simulink model "wabs_perceptionmodel_VPT_Limbic_v3_adj"  (R2014b)
settings: Solver=ode3  StartTime=0.0  StopTime=r.t(end)  FixedStep=z.dt  MaxStep=0.01  RelTol=1e-3
undefined symbols (not defined in the file or in its folder): G0, G0_hat, r, z
libraries: vrlib x3, dspinverses x1
settings Model: Creator=dpool  LastModifiedBy=fdrop
settings DataIOCC: SignalLoggingSaveFormat=ModelDataLogs
settings OptimizationCC: ExpressionDepthLimit=2147483647
settings DebuggingCC: AlgebraicLoopMsg=none  UnderspecifiedInitializationDetection=Classic  MergeDetectMultiDrivingBlocksExec=none  FcnCallInpInsideContextMsg=EnableAllAsWarning  StateNameClashWarn=warning  InitInArrayFormatMsg=none
settings SFSimCC: SimParseCustomCode=off
settings GRTTargetCC: CombineOutputUpdateFcns=off  GRTInterface=on

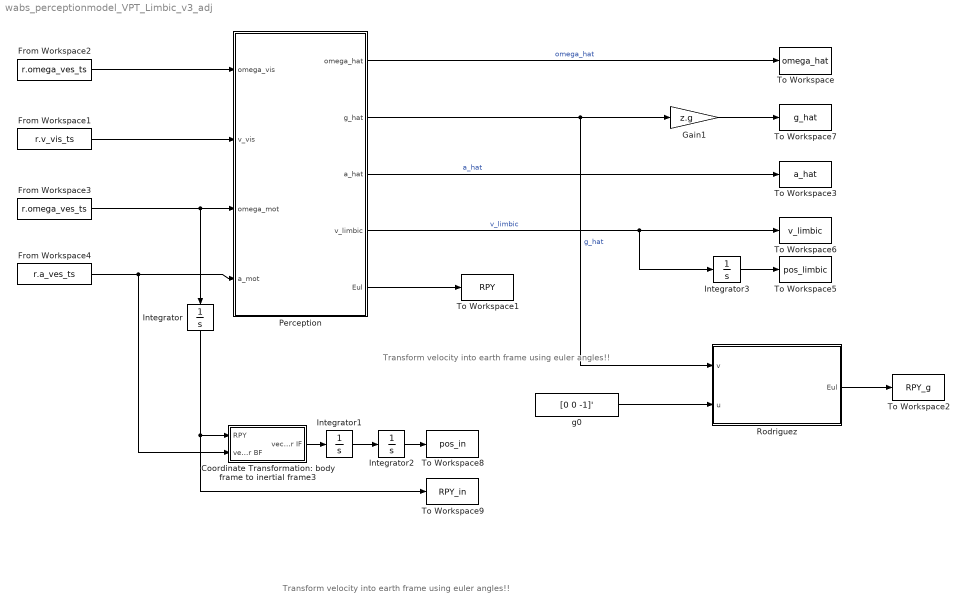
== system wabs_perceptionmodel_VPT_Limbic_v3_adj ==
  note: Transform velocity into earth frame using euler angles!!
  note: Transform velocity into earth frame using euler angles!!
  Coordinate Transformation: body frame to inertial frame3 : Subsystem
  From Workspace1 : FromWorkspace  VariableName=r.v_vis_ts  SampleTime=0
  From Workspace2 : FromWorkspace  VariableName=r.omega_ves_ts  SampleTime=0
  From Workspace3 : FromWorkspace  VariableName=r.omega_ves_ts  SampleTime=0
  From Workspace4 : FromWorkspace  VariableName=r.a_ves_ts  SampleTime=0
  Gain1 : Gain  Gain=z.g
  Integrator{,1..3} (4 alike) : Integrator
  Perception : Subsystem  mask{G0_mot=[0; 0; -1]}
      mask TypeOptions G0_mot:
      | Input Selection & Kinematics/Initial orientation,
      | motion/Value
  Rodriguez : MATLAB Function  TreatAsAtomicUnit=on
  To Workspace : ToWorkspace  VariableName=omega_hat  SampleTime=-1
  To Workspace1 : ToWorkspace  VariableName=RPY  SampleTime=-1
  To Workspace2 : ToWorkspace  VariableName=RPY_g  SampleTime=-1
  To Workspace3 : ToWorkspace  VariableName=a_hat  SampleTime=-1
  To Workspace5 : ToWorkspace  VariableName=pos_limbic  SampleTime=-1
  To Workspace6 : ToWorkspace  VariableName=v_limbic  SampleTime=-1
  To Workspace7 : ToWorkspace  VariableName=g_hat  SampleTime=-1
  To Workspace8 : ToWorkspace  VariableName=pos_in  SampleTime=-1
  To Workspace9 : ToWorkspace  VariableName=RPY_in  SampleTime=-1
  g0 : Constant  Value=[0 0 -1]'
  wires:
  Perception/1(omega_hat) -> To Workspace/1  "omega_hat"
  Perception/2(g_hat) -> Rodriguez/1(v), Gain1/1  "g_hat"
  Perception/3(a_hat) -> To Workspace3/1  "a_hat"
  Perception/4(v_limbic) -> Integrator3/1, To Workspace6/1  "v_limbic"
  Gain1/1 -> To Workspace7/1
  From Workspace4/1 -> Coordinate Transformation: body frame to inertial frame3/2(vector BF), Perception/4(a_mot)
  From Workspace3/1 -> Integrator/1, Perception/3(omega_mot)
  Perception/5(Eul) -> To Workspace1/1
  From Workspace1/1 -> Perception/2(v_vis)
  From Workspace2/1 -> Perception/1(omega_vis)
  Integrator3/1 -> To Workspace5/1
  Integrator/1 -> To Workspace9/1, Coordinate Transformation: body frame to inertial frame3/1(RPY)
  Coordinate Transformation: body frame to inertial frame3/1(vector IF) -> Integrator1/1
  Integrator1/1 -> Integrator2/1
  Integrator2/1 -> To Workspace8/1
  g0/1 -> Rodriguez/2(u)
  Rodriguez/1(Eul) -> To Workspace2/1

== system wabs_perceptionmodel_VPT_Limbic_v3_adj/Coordinate Transformation: body frame to inertial frame3 ==
  RPY : Inport
  vector BF : Inport  Port=2
  Body2Inertial : MATLAB Function  TreatAsAtomicUnit=on
  Product : Product  Multiplication=Matrix(*)  RndMeth=Zero
  vector IF : Outport
  wires:
  Body2Inertial/1(DCM) -> Product/1
  RPY/1 -> Body2Inertial/1(RPY)
  Product/1 -> vector IF/1
  vector BF/1 -> Product/2

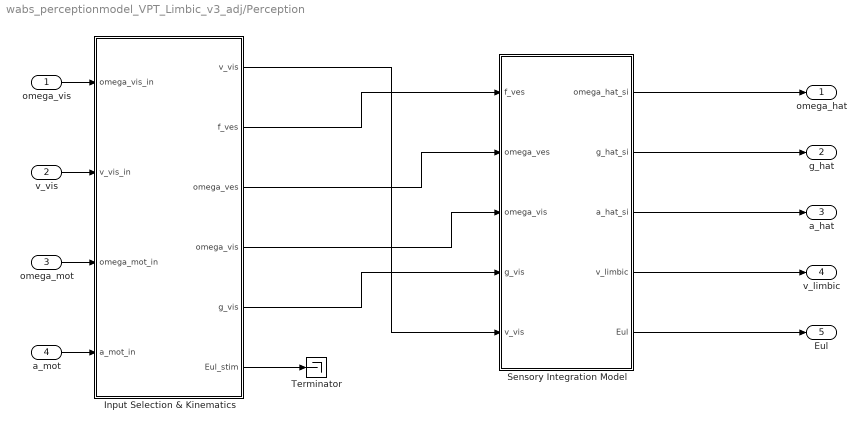
== system wabs_perceptionmodel_VPT_Limbic_v3_adj/Perception ==
  omega_vis : Inport
  v_vis : Inport  Port=2
  omega_mot : Inport  Port=3
  a_mot : Inport  Port=4
  Input Selection & Kinematics : Subsystem
  Sensory Integration Model : Subsystem
  Terminator : Terminator
  omega_hat : Outport
  g_hat : Outport  Port=2
  a_hat : Outport  Port=3
  v_limbic : Outport  Port=4
  Eul : Outport  Port=5
  wires:
  Input Selection & Kinematics/5(g_vis) -> Sensory Integration Model/4(g_vis)
  Input Selection & Kinematics/4(omega_vis) -> Sensory Integration Model/3(omega_vis)
  Input Selection & Kinematics/3(omega_ves) -> Sensory Integration Model/2(omega_ves)
  Input Selection & Kinematics/2(f_ves) -> Sensory Integration Model/1(f_ves)
  Input Selection & Kinematics/1(v_vis) -> Sensory Integration Model/5(v_vis)
  Sensory Integration Model/1(omega_hat_si) -> omega_hat/1
  omega_vis/1 -> Input Selection & Kinematics/1(omega_vis_in)
  Sensory Integration Model/2(g_hat_si) -> g_hat/1
  v_vis/1 -> Input Selection & Kinematics/2(v_vis_in)
  omega_mot/1 -> Input Selection & Kinematics/3(omega_mot_in)
  Sensory Integration Model/3(a_hat_si) -> a_hat/1
  a_mot/1 -> Input Selection & Kinematics/4(a_mot_in)
  Sensory Integration Model/4(v_limbic) -> v_limbic/1
  Sensory Integration Model/5(Eul) -> Eul/1
  Input Selection & Kinematics/6(Eul_stim) -> Terminator/1

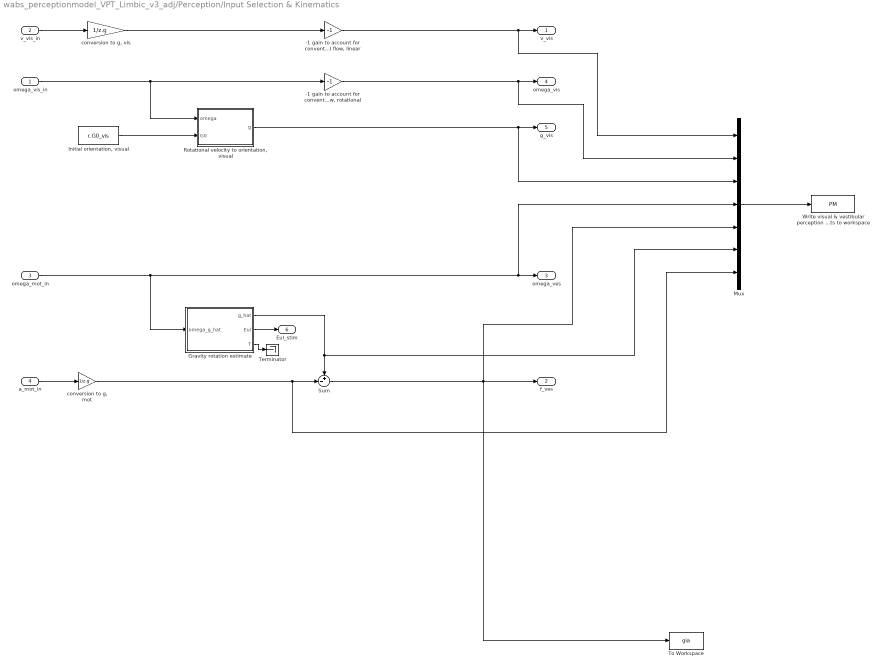
== system wabs_perceptionmodel_VPT_Limbic_v3_adj/Perception/Input Selection & Kinematics ==
  omega_vis_in : Inport
  v_vis_in : Inport  Port=2
  omega_mot_in : Inport  Port=3
  a_mot_in : Inport  Port=4
  "-1 gain to account for convention in visual flow, linear" : Gain  Gain=-1
  "-1 gain to account for convention in visual flow, rotational" : Gain  Gain=-1
  Gravity rotation estimate : Subsystem
  "Initial orientation, visual" : Constant  Value=r.G0_vis
  Mux : Mux  Inputs=7
  "Rotational velocity to orientation, visual" : Subsystem
  Sum : Sum  Inputs=+-|
  Terminator : Terminator
  To Workspace : ToWorkspace  VariableName=gia  SampleTime=-1
  Write visual & vestibular perception model inputs to workspace : ToWorkspace  VariableName=PM  SampleTime=-1
  "conversion to g, mot" : Gain  Gain=1/z.g
  "conversion to g, vis" : Gain  Gain=1/z.g
  v_vis : Outport
  f_ves : Outport  Port=2
  omega_ves : Outport  Port=3
  omega_vis : Outport  Port=4
  g_vis : Outport  Port=5
  Eul_stim : Outport  Port=6
  wires:
  a_mot_in/1 -> "conversion to g, mot"/1
  "-1 gain to account for convention in visual flow, linear"/1 -> v_vis/1, Mux/1
  v_vis_in/1 -> "conversion to g, vis"/1
  omega_vis_in/1 -> "-1 gain to account for convention in visual flow, rotational"/1, "Rotational velocity to orientation, visual"/1(omega)
  "Rotational velocity to orientation, visual"/1(g) -> g_vis/1, Mux/3
  "Initial orientation, visual"/1 -> "Rotational velocity to orientation, visual"/2(G0)
  "-1 gain to account for convention in visual flow, rotational"/1 -> omega_vis/1, Mux/2
  omega_mot_in/1 -> Gravity rotation estimate/1(omega_g_hat), omega_ves/1, Mux/4
  Gravity rotation estimate/1(g_hat) -> Sum/1, Mux/6
  Mux/1 -> Write visual & vestibular perception model inputs to workspace/1
  "conversion to g, vis"/1 -> "-1 gain to account for convention in visual flow, linear"/1
  "conversion to g, mot"/1 -> Sum/2, Mux/7
  Sum/1 -> To Workspace/1, f_ves/1, Mux/5
  Gravity rotation estimate/2(Eul) -> Eul_stim/1
  Gravity rotation estimate/3(T) -> Terminator/1

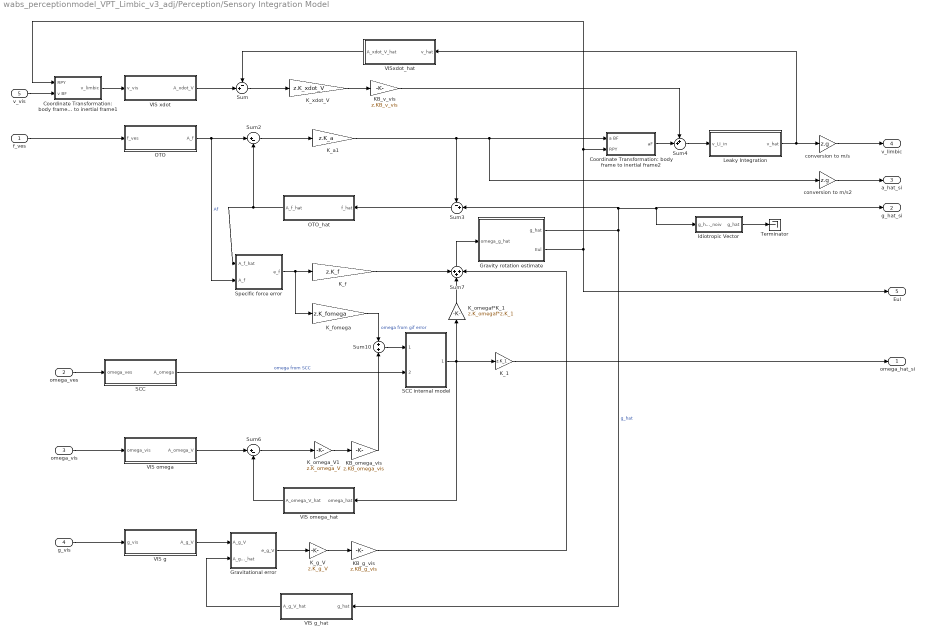
== system wabs_perceptionmodel_VPT_Limbic_v3_adj/Perception/Sensory Integration Model ==
  f_ves : Inport
  omega_ves : Inport  Port=2
  omega_vis : Inport  Port=3
  g_vis : Inport  Port=4
  v_vis : Inport  Port=5
  Coordinate Transformation: body frame to inertial frame1 : Subsystem
  Coordinate Transformation: body frame to inertial frame2 : Subsystem
  Gravitational error : Subsystem
  Gravity rotation estimate : Subsystem
  Idiotropic Vector : Subsystem
  KB_g_vis : Gain  Gain=z.KB_g_vis
  KB_omega_vis : Gain  Gain=z.KB_omega_vis
  KB_v_vis : Gain  Gain=z.KB_v_vis
  K_1 : Gain  Gain=z.K_1
  K_a1 : Gain  Gain=z.K_a
  K_f : Gain  Gain=z.K_f
  K_fomega : Gain  Gain=z.K_fomega
  K_g_V : Gain  Gain=z.K_g_V
  K_omega_V1 : Gain  Gain=z.K_omega_V
  K_omegaf*K_1 : Gain  Gain=z.K_omegaf*z.K_1
  K_xdot_V : Gain  Gain=z.K_xdot_V
  Leaky Integration : Subsystem
  OTO : Subsystem
  OTO_hat : Subsystem
  SCC : Subsystem
  SCC internal model : Subsystem
  Specific force error : Subsystem
  Sum : Sum  Inputs=-+|
  Sum10 : Sum
  Sum2 : Sum  Inputs=|+-
  Sum3 : Sum  Inputs=-+|
  Sum4 : Sum  Inputs=++|
  Sum6 : Sum  Inputs=|+-
  Sum7 : Sum  Inputs=+++
  Terminator : Terminator
  VIS g : Subsystem
  VIS g_hat : Subsystem
  VIS omega : Subsystem
  VIS omega_hat : Subsystem
  VIS xdot : Subsystem
  VISxdot_hat : Subsystem
  conversion to m/s : Gain  Gain=z.g
  conversion to m/s2 : Gain  Gain=z.g
  omega_hat_si : Outport
  g_hat_si : Outport  Port=2
  a_hat_si : Outport  Port=3
  v_limbic : Outport  Port=4
  Eul : Outport  Port=5
  wires:
  Sum2/1 -> K_a1/1
  OTO/1(A_f) -> Sum2/1, Specific force error/2(A_f)  "Af"
  Sum3/1 -> OTO_hat/1(f_hat)
  SCC/1(A_omega) -> SCC internal model/2(omega_SCC)  "omega from SCC"
  OTO_hat/1(A_f_hat) -> Sum2/2, Specific force error/1(A_f_hat)
  Gravity rotation estimate/1(g_hat) -> Idiotropic Vector/1(g_hat_noiv), g_hat_si/1, Sum3/2, VIS g_hat/1(g_hat)  "g_hat"
  Specific force error/1(e_f) -> K_f/1, K_fomega/1
  K_fomega/1 -> Sum10/1  "omega from gif error"
  VIS xdot/1(A_xdot_V) -> Sum/2
  VISxdot_hat/1(A_xdot_V_hat) -> Sum/1
  Sum/1 -> K_xdot_V/1
  K_xdot_V/1 -> KB_v_vis/1
  VIS omega/1(A_omega_V) -> Sum6/1
  Sum6/1 -> K_omega_V1/1
  VIS omega_hat/1(A_omega_V_hat) -> Sum6/2
  VIS g/1(A_g_V) -> Gravitational error/1(A_g_V)
  Gravitational error/1(e_g_V) -> K_g_V/1
  VIS g_hat/1(A_g_V_hat) -> Gravitational error/2(A_g_V_hat)
  K_1/1 -> omega_hat_si/1
  K_g_V/1 -> KB_g_vis/1
  K_omega_V1/1 -> KB_omega_vis/1
  Leaky Integration/1(v_hat) -> VISxdot_hat/1(v_hat), conversion to m/s/1
  Sum7/1 -> Gravity rotation estimate/1(omega_g_hat)
  f_ves/1 -> OTO/1(f_ves)
  omega_ves/1 -> SCC/1(omega_ves)
  omega_vis/1 -> VIS omega/1(omega_vis)
  g_vis/1 -> VIS g/1(g_vis)
  KB_g_vis/1 -> Sum7/3
  conversion to m/s/1 -> v_limbic/1
  conversion to m/s2/1 -> a_hat_si/1
  K_f/1 -> Sum7/1
  K_omegaf*K_1/1 -> Sum7/2
  K_a1/1 -> Sum3/1, Coordinate Transformation: body frame to inertial frame2/1(a BF), conversion to m/s2/1
  Idiotropic Vector/1(g_hat) -> Terminator/1
  v_vis/1 -> Coordinate Transformation: body frame to inertial frame1/2(v BF)
  Coordinate Transformation: body frame to inertial frame1/1(v_limbic) -> VIS xdot/1(v_vis)
  Gravity rotation estimate/2(Eul) -> Coordinate Transformation: body frame to inertial frame2/2(RPY), Coordinate Transformation: body frame to inertial frame1/1(RPY), Eul/1
  Coordinate Transformation: body frame to inertial frame2/1(aF) -> Sum4/2
  Sum4/1 -> Leaky Integration/1(v_LI_in)
  KB_v_vis/1 -> Sum4/1
  KB_omega_vis/1 -> Sum10/2
  Sum10/1 -> SCC internal model/1(omega_vis+GIF)
  SCC internal model/1(omega_hat) -> K_1/1, VIS omega_hat/1(omega_hat), K_omegaf*K_1/1

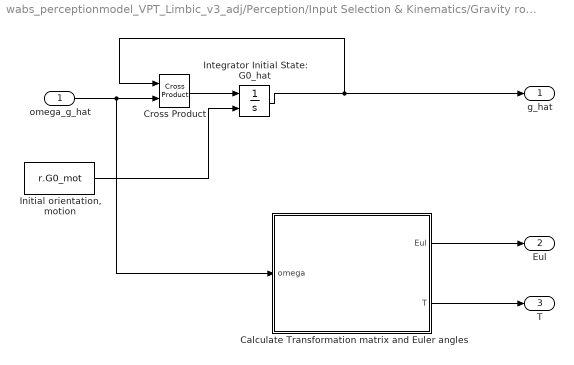
== system wabs_perceptionmodel_VPT_Limbic_v3_adj/Perception/Input Selection & Kinematics/Gravity rotation estimate ==
  omega_g_hat : Inport
  Calculate Transformation matrix and Euler angles : Subsystem
  Cross Product : vrlib/Utilities/Cross Product
  "Initial orientation, motion" : Constant  Value=r.G0_mot
  Integrator Initial State: G0_hat : Integrator  InitialConditionSource=external  InitialCondition=G0_hat
  g_hat : Outport
  Eul : Outport  Port=2
  T : Outport  Port=3
  wires:
  Integrator Initial State: G0_hat/1 -> Cross Product/1, g_hat/1
  Cross Product/1 -> Integrator Initial State: G0_hat/1
  omega_g_hat/1 -> Calculate Transformation matrix and Euler angles/1(omega), Cross Product/2
  Calculate Transformation matrix and Euler angles/1(Eul) -> Eul/1
  Calculate Transformation matrix and Euler angles/2(T) -> T/1
  "Initial orientation, motion"/1 -> Integrator Initial State: G0_hat/2

== system wabs_perceptionmodel_VPT_Limbic_v3_adj/Perception/Input Selection & Kinematics/Rotational velocity to orientation, visual ==
  omega : Inport
  G0 : Inport  Port=2
  Cross Product : vrlib/Utilities/Cross Product
  Integrator : Integrator  InitialConditionSource=external  InitialCondition=G0
  Normalize vector1 : Subsystem
  g : Outport
  wires:
  Integrator/1 -> Normalize vector1/1(G), Cross Product/1
  Cross Product/1 -> Integrator/1
  Normalize vector1/1(g) -> g/1
  omega/1 -> Cross Product/2
  G0/1 -> Integrator/2

== system wabs_perceptionmodel_VPT_Limbic_v3_adj/Perception/Sensory Integration Model/Coordinate Transformation: body frame to inertial frame1 ==
  RPY : Inport
  v BF : Inport  Port=2
  Body2Inertial : MATLAB Function  TreatAsAtomicUnit=on
  Product : Product  Multiplication=Matrix(*)  RndMeth=Zero
  v_limbic : Outport
  wires:
  Body2Inertial/1(DCM) -> Product/1
  RPY/1 -> Body2Inertial/1(RPY)
  Product/1 -> v_limbic/1
  v BF/1 -> Product/2

== system wabs_perceptionmodel_VPT_Limbic_v3_adj/Perception/Sensory Integration Model/Coordinate Transformation: body frame to inertial frame2 ==
  a BF : Inport
  RPY : Inport  Port=2
  Body2Inertial : MATLAB Function  TreatAsAtomicUnit=on
  Product : Product  Multiplication=Matrix(*)  RndMeth=Zero
  aF : Outport
  wires:
  a BF/1 -> Product/2
  Product/1 -> aF/1
  RPY/1 -> Body2Inertial/1(RPY)
  Body2Inertial/1(DCM) -> Product/1

== system wabs_perceptionmodel_VPT_Limbic_v3_adj/Perception/Sensory Integration Model/Gravitational error ==
  A_g_V : Inport
  A_g_V_hat : Inport  Port=2
  MATLAB Function : MATLAB Function  TreatAsAtomicUnit=on
  e_g_V : Outport
  wires:
  A_g_V/1 -> MATLAB Function/1(g)
  A_g_V_hat/1 -> MATLAB Function/2(g_hat)
  MATLAB Function/1(e_g) -> e_g_V/1

== system wabs_perceptionmodel_VPT_Limbic_v3_adj/Perception/Sensory Integration Model/Gravity rotation estimate ==
  omega_g_hat : Inport
  Calculate Euler angles from omega CLEANER : Subsystem
  Cross Product : vrlib/Utilities/Cross Product
  Integrator Initial State: G0_hat : Integrator  InitialCondition=r.G0_hat
  g_hat : Outport
  Eul : Outport  Port=2
  wires:
  Integrator Initial State: G0_hat/1 -> Cross Product/1, g_hat/1
  Cross Product/1 -> Integrator Initial State: G0_hat/1
  omega_g_hat/1 -> Calculate Euler angles from omega CLEANER/1(omega), Cross Product/2
  Calculate Euler angles from omega CLEANER/1(Eul) -> Eul/1

== system wabs_perceptionmodel_VPT_Limbic_v3_adj/Perception/Sensory Integration Model/Idiotropic Vector ==
  g_hat_noiv : Inport
  Idiotropic vector: constant unity vector aligned with vertical body axis : Constant  Value=r.G_iv
  K_iv : Gain  Gain=z.K_iv
  Normalize vector : Subsystem
  Sum : Sum  Inputs=++|
  g_hat : Outport
  wires:
  Normalize vector/1(g) -> g_hat/1
  Idiotropic vector: constant unity vector aligned with vertical body axis/1 -> K_iv/1
  K_iv/1 -> Sum/1
  g_hat_noiv/1 -> Sum/2
  Sum/1 -> Normalize vector/1(G)

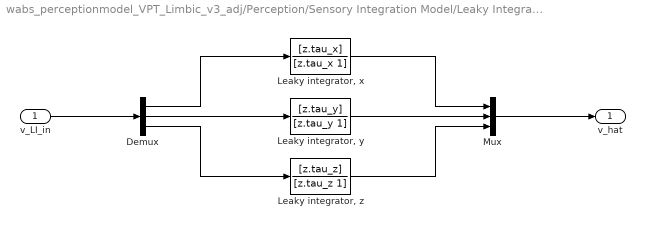
== system wabs_perceptionmodel_VPT_Limbic_v3_adj/Perception/Sensory Integration Model/Leaky Integration ==
  v_LI_in : Inport
  Demux : Demux  Outputs=3
  "Leaky integrator, x" : TransferFcn  Numerator=[z.tau_x]  Denominator=[z.tau_x 1]
  "Leaky integrator, y" : TransferFcn  Numerator=[z.tau_y]  Denominator=[z.tau_y 1]
  "Leaky integrator, z" : TransferFcn  Numerator=[z.tau_z]  Denominator=[z.tau_z 1]
  Mux : Mux  Inputs=3
  v_hat : Outport
  wires:
  v_LI_in/1 -> Demux/1
  Mux/1 -> v_hat/1
  "Leaky integrator, y"/1 -> Mux/2
  Demux/2 -> "Leaky integrator, y"/1
  Demux/1 -> "Leaky integrator, x"/1
  "Leaky integrator, x"/1 -> Mux/1
  Demux/3 -> "Leaky integrator, z"/1
  "Leaky integrator, z"/1 -> Mux/3

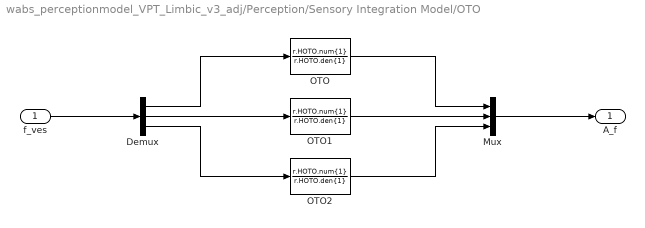
== system wabs_perceptionmodel_VPT_Limbic_v3_adj/Perception/Sensory Integration Model/OTO ==
  f_ves : Inport
  Demux : Demux  Outputs=3
  Mux : Mux  Inputs=3
  OTO : TransferFcn  Numerator=r.HOTO.num{1}  Denominator=r.HOTO.den{1}
  OTO1 : TransferFcn  Numerator=r.HOTO.num{1}  Denominator=r.HOTO.den{1}
  OTO2 : TransferFcn  Numerator=r.HOTO.num{1}  Denominator=r.HOTO.den{1}
  A_f : Outport
  wires:
  f_ves/1 -> Demux/1
  Mux/1 -> A_f/1
  OTO1/1 -> Mux/2
  Demux/2 -> OTO1/1
  Demux/1 -> OTO/1
  OTO/1 -> Mux/1
  Demux/3 -> OTO2/1
  OTO2/1 -> Mux/3

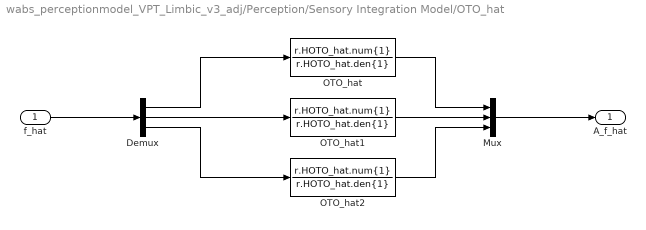
== system wabs_perceptionmodel_VPT_Limbic_v3_adj/Perception/Sensory Integration Model/OTO_hat ==
  f_hat : Inport
  Demux : Demux  Outputs=3
  Mux : Mux  Inputs=3
  OTO_hat : TransferFcn  Numerator=r.HOTO_hat.num{1}  Denominator=r.HOTO_hat.den{1}
  OTO_hat1 : TransferFcn  Numerator=r.HOTO_hat.num{1}  Denominator=r.HOTO_hat.den{1}
  OTO_hat2 : TransferFcn  Numerator=r.HOTO_hat.num{1}  Denominator=r.HOTO_hat.den{1}
  A_f_hat : Outport
  wires:
  f_hat/1 -> Demux/1
  Mux/1 -> A_f_hat/1
  OTO_hat1/1 -> Mux/2
  Demux/2 -> OTO_hat1/1
  Demux/1 -> OTO_hat/1
  OTO_hat/1 -> Mux/1
  Demux/3 -> OTO_hat2/1
  OTO_hat2/1 -> Mux/3

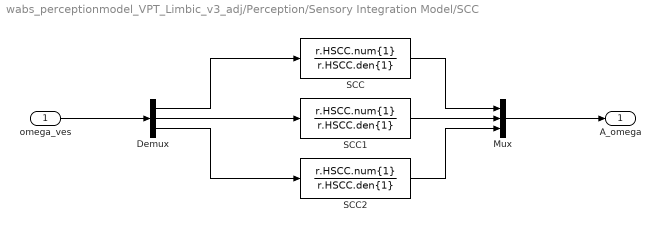
== system wabs_perceptionmodel_VPT_Limbic_v3_adj/Perception/Sensory Integration Model/SCC ==
  omega_ves : Inport
  Demux : Demux  Outputs=3
  Mux : Mux  Inputs=3
  SCC : TransferFcn  Numerator=r.HSCC.num{1}  Denominator=r.HSCC.den{1}
  SCC1 : TransferFcn  Numerator=r.HSCC.num{1}  Denominator=r.HSCC.den{1}
  SCC2 : TransferFcn  Numerator=r.HSCC.num{1}  Denominator=r.HSCC.den{1}
  A_omega : Outport
  wires:
  omega_ves/1 -> Demux/1
  Mux/1 -> A_omega/1
  SCC1/1 -> Mux/2
  Demux/2 -> SCC1/1
  Demux/1 -> SCC/1
  SCC/1 -> Mux/1
  Demux/3 -> SCC2/1
  SCC2/1 -> Mux/3

== system wabs_perceptionmodel_VPT_Limbic_v3_adj/Perception/Sensory Integration Model/SCC internal model ==
  omega_vis+GIF : Inport
  omega_SCC : Inport  Port=2
  K_omega : Gain  Gain=z.K_omega
  SCC_hat : Subsystem
  Sum5 : Sum
  omega_hat : Outport
  wires:
  omega_SCC/1 -> K_omega/1
  SCC_hat/1(A_omega_hat) -> omega_hat/1
  omega_vis+GIF/1 -> Sum5/1
  K_omega/1 -> Sum5/2
  Sum5/1 -> SCC_hat/1(omega_hat)

== system wabs_perceptionmodel_VPT_Limbic_v3_adj/Perception/Sensory Integration Model/Specific force error ==
  A_f_hat : Inport
  A_f : Inport  Port=2
  Specific force rotation error : MATLAB Function  TreatAsAtomicUnit=on
  e_f : Outport
  wires:
  Specific force rotation error/1(ef) -> e_f/1
  A_f/1 -> Specific force rotation error/1(af)
  A_f_hat/1 -> Specific force rotation error/2(af_hat)

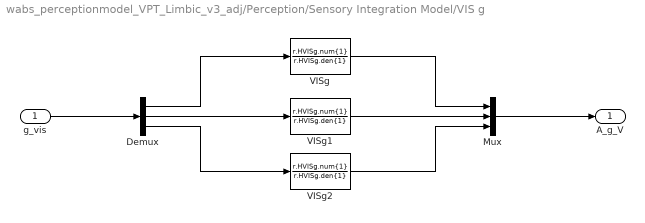
== system wabs_perceptionmodel_VPT_Limbic_v3_adj/Perception/Sensory Integration Model/VIS g ==
  g_vis : Inport
  Demux : Demux  Outputs=3
  Mux : Mux  Inputs=3
  VISg : TransferFcn  Numerator=r.HVISg.num{1}  Denominator=r.HVISg.den{1}
  VISg1 : TransferFcn  Numerator=r.HVISg.num{1}  Denominator=r.HVISg.den{1}
  VISg2 : TransferFcn  Numerator=r.HVISg.num{1}  Denominator=r.HVISg.den{1}
  A_g_V : Outport
  wires:
  g_vis/1 -> Demux/1
  Mux/1 -> A_g_V/1
  VISg1/1 -> Mux/2
  Demux/2 -> VISg1/1
  Demux/1 -> VISg/1
  VISg/1 -> Mux/1
  Demux/3 -> VISg2/1
  VISg2/1 -> Mux/3

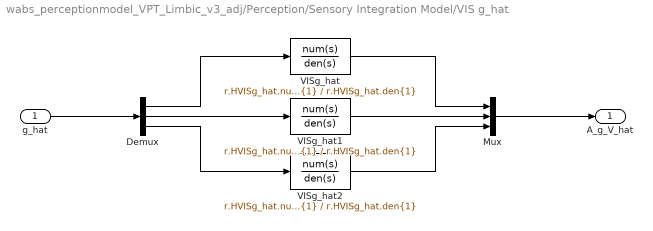
== system wabs_perceptionmodel_VPT_Limbic_v3_adj/Perception/Sensory Integration Model/VIS g_hat ==
  g_hat : Inport
  Demux : Demux  Outputs=3
  Mux : Mux  Inputs=3
  VISg_hat : TransferFcn  Numerator=r.HVISg_hat.num{1}  Denominator=r.HVISg_hat.den{1}
  VISg_hat1 : TransferFcn  Numerator=r.HVISg_hat.num{1}  Denominator=r.HVISg_hat.den{1}
  VISg_hat2 : TransferFcn  Numerator=r.HVISg_hat.num{1}  Denominator=r.HVISg_hat.den{1}
  A_g_V_hat : Outport
  wires:
  g_hat/1 -> Demux/1
  Mux/1 -> A_g_V_hat/1
  VISg_hat1/1 -> Mux/2
  Demux/2 -> VISg_hat1/1
  Demux/1 -> VISg_hat/1
  VISg_hat/1 -> Mux/1
  Demux/3 -> VISg_hat2/1
  VISg_hat2/1 -> Mux/3

== system wabs_perceptionmodel_VPT_Limbic_v3_adj/Perception/Sensory Integration Model/VIS omega ==
  omega_vis : Inport
  Demux : Demux  Outputs=3
  Mux : Mux  Inputs=3
  VISomega : TransferFcn  Numerator=r.HVISomega.num{1}  Denominator=r.HVISomega.den{1}
  VISomega1 : TransferFcn  Numerator=r.HVISomega.num{1}  Denominator=r.HVISomega.den{1}
  VISomega2 : TransferFcn  Numerator=r.HVISomega.num{1}  Denominator=r.HVISomega.den{1}
  A_omega_V : Outport
  wires:
  omega_vis/1 -> Demux/1
  Mux/1 -> A_omega_V/1
  VISomega1/1 -> Mux/2
  Demux/2 -> VISomega1/1
  Demux/1 -> VISomega/1
  VISomega/1 -> Mux/1
  Demux/3 -> VISomega2/1
  VISomega2/1 -> Mux/3

== system wabs_perceptionmodel_VPT_Limbic_v3_adj/Perception/Sensory Integration Model/VIS omega_hat ==
  omega_hat : Inport
  Demux : Demux  Outputs=3
  Mux : Mux  Inputs=3
  VISomega_hat : TransferFcn  Numerator=r.HVISomega_hat.num{1}  Denominator=r.HVISomega_hat.den{1}
  VISomega_hat1 : TransferFcn  Numerator=r.HVISomega_hat.num{1}  Denominator=r.HVISomega_hat.den{1}
  VISomega_hat2 : TransferFcn  Numerator=r.HVISomega_hat.num{1}  Denominator=r.HVISomega_hat.den{1}
  A_omega_V_hat : Outport
  wires:
  omega_hat/1 -> Demux/1
  Mux/1 -> A_omega_V_hat/1
  VISomega_hat1/1 -> Mux/2
  Demux/2 -> VISomega_hat1/1
  Demux/1 -> VISomega_hat/1
  VISomega_hat/1 -> Mux/1
  Demux/3 -> VISomega_hat2/1
  VISomega_hat2/1 -> Mux/3

== system wabs_perceptionmodel_VPT_Limbic_v3_adj/Perception/Sensory Integration Model/VIS xdot ==
  v_vis : Inport
  Demux : Demux  Outputs=3
  Mux : Mux  Inputs=3
  VISxdot : TransferFcn  Numerator=r.HVISxdot.num{1}  Denominator=r.HVISxdot.den{1}
  VISxdot1 : TransferFcn  Numerator=r.HVISxdot.num{1}  Denominator=r.HVISxdot.den{1}
  VISxdot2 : TransferFcn  Numerator=r.HVISxdot.num{1}  Denominator=r.HVISxdot.den{1}
  A_xdot_V : Outport
  wires:
  v_vis/1 -> Demux/1
  Mux/1 -> A_xdot_V/1
  VISxdot1/1 -> Mux/2
  Demux/2 -> VISxdot1/1
  Demux/1 -> VISxdot/1
  VISxdot/1 -> Mux/1
  Demux/3 -> VISxdot2/1
  VISxdot2/1 -> Mux/3

== system wabs_perceptionmodel_VPT_Limbic_v3_adj/Perception/Sensory Integration Model/VISxdot_hat ==
  v_hat : Inport
  Demux : Demux  Outputs=3
  Mux : Mux  Inputs=3
  VISxdot_hat : TransferFcn  Numerator=r.HVISxdot_hat.num{1}  Denominator=r.HVISxdot_hat.den{1}
  VISxdot_hat1 : TransferFcn  Numerator=r.HVISxdot_hat.num{1}  Denominator=r.HVISxdot_hat.den{1}
  VISxdot_hat2 : TransferFcn  Numerator=r.HVISxdot_hat.num{1}  Denominator=r.HVISxdot_hat.den{1}
  A_xdot_V_hat : Outport
  wires:
  v_hat/1 -> Demux/1
  Mux/1 -> A_xdot_V_hat/1
  VISxdot_hat1/1 -> Mux/2
  Demux/2 -> VISxdot_hat1/1
  Demux/1 -> VISxdot_hat/1
  VISxdot_hat/1 -> Mux/1
  Demux/3 -> VISxdot_hat2/1
  VISxdot_hat2/1 -> Mux/3

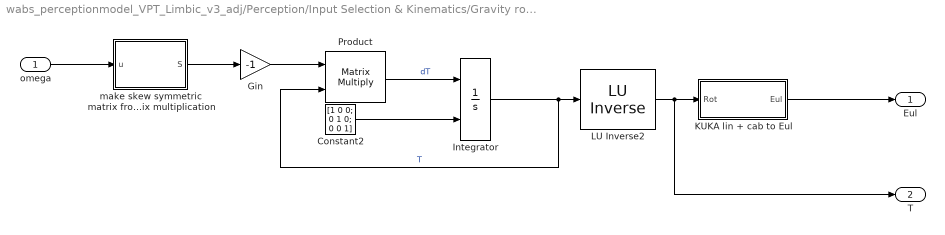
== system wabs_perceptionmodel_VPT_Limbic_v3_adj/Perception/Input Selection & Kinematics/Gravity rotation estimate/Calculate Transformation matrix and Euler angles ==
  omega : Inport
  " LU Inverse2" : dspinverses/ LU Inverse
  Constant2 : Constant  Value=[1 0 0; 0 1 0; 0 0 1]
  Gin : Gain  Gain=-1
  Integrator : Integrator  InitialConditionSource=external  InitialCondition=[1 0 0; 0 1 0; 0 0 1]
  KUKA lin + cab to Eul : Subsystem  AncestorBlock=KUKA_Control_libs/KUKA lin + cab to Eul
  Product : Product  Multiplication=Matrix(*)
  make skew symmetric matrix from omega for matrix multiplication : MATLAB Function  TreatAsAtomicUnit=on
  Eul : Outport
  T : Outport  Port=2
  wires:
  Integrator/1 -> " LU Inverse2"/1, Product/2  "T"
  KUKA lin + cab to Eul/1(Eul) -> Eul/1
  make skew symmetric matrix from omega for matrix multiplication/1(S) -> Gin/1
  Product/1 -> Integrator/1  "dT"
  omega/1 -> make skew symmetric matrix from omega for matrix multiplication/1(u)
  Constant2/1 -> Integrator/2
  Gin/1 -> Product/1
  " LU Inverse2"/1 -> T/1, KUKA lin + cab to Eul/1(Rot)

== system wabs_perceptionmodel_VPT_Limbic_v3_adj/Perception/Input Selection & Kinematics/Rotational velocity to orientation, visual/Normalize vector1 ==
  G : Inport
  Mux3 : Mux  Inputs=3
  "Normalize, u(1)" : Fcn  Expr=u(1)/sqrt(u(1)^2+u(2)^2+u(3)^2)
  "Normalize, u(2" : Fcn  Expr=u(2)/sqrt(u(1)^2+u(2)^2+u(3)^2)
  "Normalize, u(3)" : Fcn  Expr=u(3)/sqrt(u(1)^2+u(2)^2+u(3)^2)
  g : Outport
  wires:
  Mux3/1 -> g/1
  "Normalize, u(3)"/1 -> Mux3/3
  "Normalize, u(2"/1 -> Mux3/2
  "Normalize, u(1)"/1 -> Mux3/1
  G/1 -> "Normalize, u(2"/1, "Normalize, u(1)"/1, "Normalize, u(3)"/1

== system wabs_perceptionmodel_VPT_Limbic_v3_adj/Perception/Sensory Integration Model/Gravity rotation estimate/Calculate Euler angles from omega CLEANER ==
  note: Here we solve the equation dR/dt = S*R, where S is the skew symmetric matrix of omega
      | (This is the same as solving S = dR/dt * transpose(R), becuse transpose(R) *R = I )
      |
      | R is the rotation matrix that rotates the unit vectors of the head frame from a certain start orientation into a new orientation.
      | It thus expresses the transformation of a vector from head to world frame.
  omega : Inport
  Constant2 : Constant  Value=[1 0 0; 0 1 0; 0 0 1]
  Integrator : Integrator  InitialConditionSource=external  InitialCondition=[1 0 0; 0 1 0; 0 0 1]
  KUKA lin + cab to Eul : Subsystem  AncestorBlock=KUKA_Control_libs/KUKA lin + cab to Eul
  Product : Product  Multiplication=Matrix(*)
  make skew symmetric matrix from omega for matrix multiplication : MATLAB Function  TreatAsAtomicUnit=on
  Eul : Outport
  wires:
  Integrator/1 -> KUKA lin + cab to Eul/1(Rot), Product/2  "T"
  KUKA lin + cab to Eul/1(Eul) -> Eul/1
  Product/1 -> Integrator/1  "dT"
  Constant2/1 -> Integrator/2
  omega/1 -> make skew symmetric matrix from omega for matrix multiplication/1(u)
  make skew symmetric matrix from omega for matrix multiplication/1(S) -> Product/1

== system wabs_perceptionmodel_VPT_Limbic_v3_adj/Perception/Sensory Integration Model/Idiotropic Vector/Normalize vector ==
  G : Inport
  Mux3 : Mux  Inputs=3
  "Normalize, u(1)" : Fcn  Expr=u(1)/sqrt(u(1)^2+u(2)^2+u(3)^2)
  "Normalize, u(2" : Fcn  Expr=u(2)/sqrt(u(1)^2+u(2)^2+u(3)^2)
  "Normalize, u(3)" : Fcn  Expr=u(3)/sqrt(u(1)^2+u(2)^2+u(3)^2)
  g : Outport
  wires:
  Mux3/1 -> g/1
  "Normalize, u(3)"/1 -> Mux3/3
  "Normalize, u(2"/1 -> Mux3/2
  "Normalize, u(1)"/1 -> Mux3/1
  G/1 -> "Normalize, u(2"/1, "Normalize, u(1)"/1, "Normalize, u(3)"/1

== system wabs_perceptionmodel_VPT_Limbic_v3_adj/Perception/Sensory Integration Model/SCC internal model/SCC_hat ==
  omega_hat : Inport
  Demux : Demux  Outputs=3
  Mux : Mux  Inputs=3
  SCC_hat : TransferFcn  Numerator=r.HSCC_hat.num{1}  Denominator=z.K_omega * r.HSCC_hat.num{1} + r.HSCC_hat.den{1}
  SCC_hat1 : TransferFcn  Numerator=r.HSCC_hat.num{1}  Denominator=z.K_omega * r.HSCC_hat.num{1} + r.HSCC_hat.den{1}
  SCC_hat2 : TransferFcn  Numerator=r.HSCC_hat.num{1}  Denominator=z.K_omega * r.HSCC_hat.num{1} + r.HSCC_hat.den{1}
  A_omega_hat : Outport
  wires:
  SCC_hat2/1 -> Mux/3
  Demux/3 -> SCC_hat2/1
  SCC_hat/1 -> Mux/1
  Demux/1 -> SCC_hat/1
  Demux/2 -> SCC_hat1/1
  SCC_hat1/1 -> Mux/2
  Mux/1 -> A_omega_hat/1
  omega_hat/1 -> Demux/1

== system wabs_perceptionmodel_VPT_Limbic_v3_adj/Perception/Input Selection & Kinematics/Gravity rotation estimate/Calculate Transformation matrix and Euler angles/KUKA lin + cab to Eul ==
  Rot : Inport
  KUKA lin + cab to Eul : MATLAB Function  TreatAsAtomicUnit=on
  Eul : Outport
  wires:
  Rot/1 -> KUKA lin + cab to Eul/1(Rot)
  KUKA lin + cab to Eul/1(Eul) -> Eul/1

== system wabs_perceptionmodel_VPT_Limbic_v3_adj/Perception/Sensory Integration Model/Gravity rotation estimate/Calculate Euler angles from omega CLEANER/KUKA lin + cab to Eul ==
  Rot : Inport
  KUKA lin + cab to Eul : MATLAB Function  TreatAsAtomicUnit=on
  Eul : Outport
  wires:
  Rot/1 -> KUKA lin + cab to Eul/1(Rot)
  KUKA lin + cab to Eul/1(Eul) -> Eul/1

== matlab function wabs_perceptionmodel_VPT_Limbic_v3_adj/Perception/Sensory Integration Model/Specific force error/Specific force rotation error ==
  data: af input; ef output; af_hat input
function ef = fcn(af, af_hat)

% check vector lengths
if length(af) ~= 3
    error(['Vector af length not equal to 3, but ' num2str(length(af)) '!!!'])
end
if length(af_hat) ~= 3
    error(['Vector af_hat length not equal to 3, but ' num2str(length(af_hat)) '!!!'])
end

% calculate vector magnitudes
abs_af     = sqrt(sum(af.^2));
abs_af_hat = sqrt(sum(af_hat.^2));

% calculate gravitational error length
abs_ef = abs(acos(complex(dot(af/abs_af, af_hat/abs_af_hat))));

% calculate cross product and its absolute value
cross_af_afhat     = cross(af,af_hat);
abs_cross_af_afhat = sqrt(sum(cross_af_afhat.^2));

% calculate gravitational error vector
if abs_cross_af_afhat == 0
    ef = [0 0 0].';
else
    ef = cross_af_afhat / abs_cross_af_afhat * abs_ef;
end

== matlab function wabs_perceptionmodel_VPT_Limbic_v3_adj/Perception/Sensory Integration Model/Gravitational error/MATLAB Function ==
  data: g input; e_g output; g_hat input
function e_g = fcn(g, g_hat)

% check vector lengths
if length(g) ~= 3
    error(['Vector alpha_g_V length not equal to 3, but ' num2str(length(g)) '!!!'])
end
if length(g_hat) ~= 3
    error(['Vector alpha_g_V_hat length not equal to 3, but ' num2str(length(g_hat)) '!!!'])
end

% calculate vector magnitudes
abs_g     = sqrt(sum(g.^2));
abs_g_hat = sqrt(sum(g_hat.^2));

% calculate gravitational error length
abs_egV = abs(acos(complex(dot(g/abs_g, g_hat/abs_g_hat))));

% calculate cross product and its absolute value
cross_g_ghat     = cross(g,g_hat);
abs_cross_g_ghat = sqrt(sum(cross_g_ghat.^2));

% calculate gravitational error vector
if abs_cross_g_ghat == 0
    e_g = [0 0 0].';
else
    e_g = cross_g_ghat / abs_cross_g_ghat * abs_egV;
end

== matlab function wabs_perceptionmodel_VPT_Limbic_v3_adj/Perception/Input Selection & Kinematics/Gravity rotation estimate/Calculate Transformation matrix and Euler angles/KUKA lin + cab to Eul/KUKA lin + cab to Eul ==
  data: Eul output; Rot input
function Eul = fcn(Rot)


Eul = [ atan2(Rot(3,2),Rot(3,3));
        atan2(-Rot(3,1),sqrt(Rot(3,2)^2+Rot(3,3)^2));
        atan2(Rot(2,1),Rot(1,1))];
% 
% Eul = [ atan(Rot(3,2)/Rot(3,3));
%         atan(-Rot(3,1)/(sqrt(Rot(3,2)^2+Rot(3,3)^2)));
%         atan(Rot(2,1)/Rot(1,1))];

== matlab function wabs_perceptionmodel_VPT_Limbic_v3_adj/Perception/Input Selection & Kinematics/Gravity rotation estimate/Calculate Transformation matrix and Euler angles/make skew symmetric matrix from omega for matrix multiplication ==
  data: u input; S output
function S = fcn(u)
%#codegen
S = [0 -u(3) u(2); u(3) 0 -u(1); -u(2) u(1) 0];

== matlab function wabs_perceptionmodel_VPT_Limbic_v3_adj/Coordinate Transformation: body frame to inertial frame3/Body2Inertial ==
  data: RPY input; DCM output
function DCM = BF2IF(RPY)
% This block supports the Embedded MATLAB subset.
% See the help menu for details. 

r = RPY(1);
p = RPY(2);
y = RPY(3);
RPYrot = [ cos(y)*cos(p)  cos(y)*sin(p)*sin(r)-sin(y)*cos(r)  cos(y)*sin(p)*cos(r)+sin(y)*sin(r);
          sin(y)*cos(p)  sin(y)*sin(p)*sin(r)+cos(y)*cos(r)  sin(y)*sin(p)*cos(r)-cos(y)*sin(r);
             -sin(p)                  cos(p)*sin(r)                      cos(p)*cos(r)];

DCM = RPYrot;

== matlab function wabs_perceptionmodel_VPT_Limbic_v3_adj/Perception/Sensory Integration Model/Coordinate Transformation: body frame to inertial frame2/Body2Inertial ==
  data: RPY input; DCM output
function DCM = BF2IF(RPY)
% This block supports the Embedded MATLAB subset.
% See the help menu for details. 

r = RPY(1);
p = RPY(2);
y = RPY(3);
RPYrot = [ cos(y)*cos(p)  cos(y)*sin(p)*sin(r)-sin(y)*cos(r)  cos(y)*sin(p)*cos(r)+sin(y)*sin(r);
          sin(y)*cos(p)  sin(y)*sin(p)*sin(r)+cos(y)*cos(r)  sin(y)*sin(p)*cos(r)-cos(y)*sin(r);
             -sin(p)                  cos(p)*sin(r)                      cos(p)*cos(r)];

DCM = RPYrot;

== matlab function wabs_perceptionmodel_VPT_Limbic_v3_adj/Perception/Sensory Integration Model/Gravity rotation estimate/Calculate Euler angles from omega CLEANER/KUKA lin + cab to Eul/KUKA lin + cab to Eul ==
  data: Eul output; Rot input
function Eul = fcn(Rot)


Eul = [ atan2(Rot(3,2),Rot(3,3));
        atan2(-Rot(3,1),sqrt(Rot(3,2)^2+Rot(3,3)^2));
        atan2(Rot(2,1),Rot(1,1))];
    
    
    
% 
% Eul = [ atan(Rot(3,2)/Rot(3,3));
%         atan(-Rot(3,1)/(sqrt(Rot(3,2)^2+Rot(3,3)^2)));
%         atan(Rot(2,1)/Rot(1,1))];

== matlab function wabs_perceptionmodel_VPT_Limbic_v3_adj/Rodriguez ==
  data: v input; u input; Eul output
function Eul  = fcn(v, u)

epsilon = 0.1 * pi/180;

%%%%%%%%%%%%%%%%%%%%%%%%%%%%%
%Method 1: Rodigues formula
%%%%%%%%%%%%%%%%%%%%%%%%%%%%%

% find the axis and the angle that rotates vector u to v

n = cross(u,v) / norm(cross(u,v)); % normalized normal vector 

% angle between the 2 vectors
alpha = acos( dot(u,v) / ( norm(u) * norm(v) ) );


% deal with case where alpha approches 180: find a vector that is
% orthogonal to a 

if pi - alpha <= epsilon
    idx = find(u==min(u), 1, 'first'); % find idx where u is miminal
    I = eye(3);
    n = I(:,idx(1));
end
    
% Determine skew symmetric matrix
nx =  GetSkewSymmetric(n);

% % Method 1a: Rodrigues
% I = eye(3); %identity matrix
% R = I + sin(alpha)*nx + (1-cos(alpha)) * nx^2; % NB in the powerterm not elementwise!
% Eul = Rot2Eul(R);

% Method 1b: Using Matrix exponential (command "expm"!!)

% deal with very small angles
if alpha <= epsilon
    R = eye(3);
else
    R = expm(nx*alpha);
end
   
Eul = Rot2Eul(R');

end % codegen



%%%%%%%%%%%%%% FUNCTIONS %%%%%%%%%%%%%%%%%%%%%%%%%%%%%%

function S = GetSkewSymmetric(u)
S = [0 -u(3) u(2); u(3) 0 -u(1); -u(2) u(1) 0];
end

function Eul = Rot2Eul(Rot)
Eul = [ atan2(Rot(3,2),Rot(3,3));
        atan2(-Rot(3,1),sqrt(Rot(3,2)^2+Rot(3,3)^2));
        atan2(Rot(2,1),Rot(1,1))];
end

== matlab function wabs_perceptionmodel_VPT_Limbic_v3_adj/Perception/Sensory Integration Model/Coordinate Transformation: body frame to inertial frame1/Body2Inertial ==
  data: RPY input; DCM output
function DCM = BF2IF(RPY)
% This block supports the Embedded MATLAB subset.
% See the help menu for details. 

r = RPY(1);
p = RPY(2);
y = RPY(3);
RPYrot = [ cos(y)*cos(p)  cos(y)*sin(p)*sin(r)-sin(y)*cos(r)  cos(y)*sin(p)*cos(r)+sin(y)*sin(r);
          sin(y)*cos(p)  sin(y)*sin(p)*sin(r)+cos(y)*cos(r)  sin(y)*sin(p)*cos(r)-cos(y)*sin(r);
             -sin(p)                  cos(p)*sin(r)                      cos(p)*cos(r)];

DCM = RPYrot;

== matlab function wabs_perceptionmodel_VPT_Limbic_v3_adj/Perception/Sensory Integration Model/Gravity rotation estimate/Calculate Euler angles from omega CLEANER/make skew symmetric matrix from omega for matrix multiplication ==
  data: u input; S output
function S = fcn(u)
%#codegen
S = [0 -u(3) u(2); u(3) 0 -u(1); -u(2) u(1) 0];
